simulink model "Helicopter_Non_linear_ex"  (R2018a)
settings: Solver=FixedStepAuto  StartTime=4371.0  StopTime=5862  FixedStep=0.2  RelTol=1e-3
model workspace (MAT data in the model file):
  tp6fc6b471_771e_48c6_9efd_2679798d0b46.time = 0
  tp6fc6b471_771e_48c6_9efd_2679798d0b46.signals(1).values = -0.785398163397
  tp6fc6b471_771e_48c6_9efd_2679798d0b46.signals(1).dimensions = 1
  tp6fc6b471_771e_48c6_9efd_2679798d0b46.signals(1).label = 'CSTATE'
  tp6fc6b471_771e_48c6_9efd_2679798d0b46.signals(1).blockName = 'Helicopter_Non_linear_ex/Integrator'
  tp6fc6b471_771e_48c6_9efd_2679798d0b46.signals(1).stateName = ''
  tp6fc6b471_771e_48c6_9efd_2679798d0b46.signals(1).inReferencedModel = 0
  tp6fc6b471_771e_48c6_9efd_2679798d0b46.signals(1).sampleTime = [0 0]
  tp6fc6b471_771e_48c6_9efd_2679798d0b46.signals(2).values = 1.21691147844
  tp6fc6b471_771e_48c6_9efd_2679798d0b46.signals(2).dimensions = 1
  tp6fc6b471_771e_48c6_9efd_2679798d0b46.signals(2).label = 'CSTATE'
  tp6fc6b471_771e_48c6_9efd_2679798d0b46.signals(2).blockName = 'Helicopter_Non_linear_ex/Integrator1'
  tp6fc6b471_771e_48c6_9efd_2679798d0b46.signals(2).stateName = ''
  tp6fc6b471_771e_48c6_9efd_2679798d0b46.signals(2).inReferencedModel = 0
  tp6fc6b471_771e_48c6_9efd_2679798d0b46.signals(2).sampleTime = [0 0]
  tp6fc6b471_771e_48c6_9efd_2679798d0b46.signals(3).values = 1
  tp6fc6b471_771e_48c6_9efd_2679798d0b46.signals(3).dimensions = 1
  tp6fc6b471_771e_48c6_9efd_2679798d0b46.signals(3).label = 'CSTATE'
  tp6fc6b471_771e_48c6_9efd_2679798d0b46.signals(3).blockName = 'Helicopter_Non_linear_ex/Integrator2'
  tp6fc6b471_771e_48c6_9efd_2679798d0b46.signals(3).stateName = ''
  tp6fc6b471_771e_48c6_9efd_2679798d0b46.signals(3).inReferencedModel = 0
  tp6fc6b471_771e_48c6_9efd_2679798d0b46.signals(3).sampleTime = [0 0]
  tp6fc6b471_771e_48c6_9efd_2679798d0b46.signals(4).values = -0.483892496659
  tp6fc6b471_771e_48c6_9efd_2679798d0b46.signals(4).dimensions = 1
  tp6fc6b471_771e_48c6_9efd_2679798d0b46.signals(4).label = 'CSTATE'
  tp6fc6b471_771e_48c6_9efd_2679798d0b46.signals(4).blockName = 'Helicopter_Non_linear_ex/Integrator3'
  tp6fc6b471_771e_48c6_9efd_2679798d0b46.signals(4).stateName = ''
  tp6fc6b471_771e_48c6_9efd_2679798d0b46.signals(4).inReferencedModel = 0
  tp6fc6b471_771e_48c6_9efd_2679798d0b46.signals(4).sampleTime = [0 0]
  tp898a3b84_44fb_438a_a53f_dc007c783af6.time = 310
  tp898a3b84_44fb_438a_a53f_dc007c783af6.signals(1).values = -4.83010382755
  tp898a3b84_44fb_438a_a53f_dc007c783af6.signals(1).dimensions = 1
  tp898a3b84_44fb_438a_a53f_dc007c783af6.signals(1).label = 'CSTATE'
  tp898a3b84_44fb_438a_a53f_dc007c783af6.signals(1).blockName = 'Helicopter_Non_linear_ex/Integrator'
  tp898a3b84_44fb_438a_a53f_dc007c783af6.signals(1).stateName = ''
  tp898a3b84_44fb_438a_a53f_dc007c783af6.signals(1).inReferencedModel = 0
  tp898a3b84_44fb_438a_a53f_dc007c783af6.signals(1).sampleTime = [0 0]
  tp898a3b84_44fb_438a_a53f_dc007c783af6.signals(2).values = 1.21691147844
  tp898a3b84_44fb_438a_a53f_dc007c783af6.signals(2).dimensions = 1
  tp898a3b84_44fb_438a_a53f_dc007c783af6.signals(2).label = 'CSTATE'
  tp898a3b84_44fb_438a_a53f_dc007c783af6.signals(2).blockName = 'Helicopter_Non_linear_ex/Integrator1'
  tp898a3b84_44fb_438a_a53f_dc007c783af6.signals(2).stateName = ''
  tp898a3b84_44fb_438a_a53f_dc007c783af6.signals(2).inReferencedModel = 0
  tp898a3b84_44fb_438a_a53f_dc007c783af6.signals(2).sampleTime = [0 0]
  tp898a3b84_44fb_438a_a53f_dc007c783af6.signals(3).values = 4.83651296756
  tp898a3b84_44fb_438a_a53f_dc007c783af6.signals(3).dimensions = 1
  tp898a3b84_44fb_438a_a53f_dc007c783af6.signals(3).label = 'CSTATE'
  tp898a3b84_44fb_438a_a53f_dc007c783af6.signals(3).blockName = 'Helicopter_Non_linear_ex/Integrator2'
  tp898a3b84_44fb_438a_a53f_dc007c783af6.signals(3).stateName = ''
  tp898a3b84_44fb_438a_a53f_dc007c783af6.signals(3).inReferencedModel = 0
  tp898a3b84_44fb_438a_a53f_dc007c783af6.signals(3).sampleTime = [0 0]
  tp898a3b84_44fb_438a_a53f_dc007c783af6.signals(4).values = -0.483892496659
  tp898a3b84_44fb_438a_a53f_dc007c783af6.signals(4).dimensions = 1
  tp898a3b84_44fb_438a_a53f_dc007c783af6.signals(4).label = 'CSTATE'
  tp898a3b84_44fb_438a_a53f_dc007c783af6.signals(4).blockName = 'Helicopter_Non_linear_ex/Integrator3'
  tp898a3b84_44fb_438a_a53f_dc007c783af6.signals(4).stateName = ''
  tp898a3b84_44fb_438a_a53f_dc007c783af6.signals(4).inReferencedModel = 0
  tp898a3b84_44fb_438a_a53f_dc007c783af6.signals(4).sampleTime = [0 0]
values from neighbouring files (symbols this model uses):
  Bp = 0.01    [Helicopter_Values.m]
  By = 0.08    [Helicopter_Values.m]
  g = 9.81    [Helicopter_Values.m]
  jeqp = 0.0172    [Helicopter_Values.m]
  jeqy = 0.021    [Helicopter_Values.m]
  kpp = 0.0556    [Helicopter_Values.m]
  kpy = 0.005    [Helicopter_Values.m]
  kyp = 0.15    [Helicopter_Values.m]
  kyy = 0.21084    [Helicopter_Values.m]
  lcm = 0.015    [Helicopter_Values.m]
  mheli = 0.479    [Helicopter_Values.m]
undefined symbols (not defined in the file or in its folder): d2r
settings Model: Creator=pacoa  LastModifiedBy=pacoa
settings DataIOCC: ExternalInput=tp035601c0_6253_4429_837b_fd395f9a609e(1),tp035601c0_6253_4429_837b_fd395f9a609e(2),tp035601c0_6253_4429_837b_fd395f9a609e(3),tp035601c0_6253_4429_837b_fd395f9a609e(4),tp035601c0_6253_4429_837b_fd395f9a609e(5),tp035601c0_6253_4429_837b_fd395f9a609e(6)  InitialState=tp6fc6b471_771e_48c6_9efd_2679798d0b46  ReturnWorkspaceOutputs=on  OutputOption=AdditionalOutputTimes  OutputTimes=SDO_OutputTimes  ReturnWorkspaceOutputsName=SDOSimTest_Log

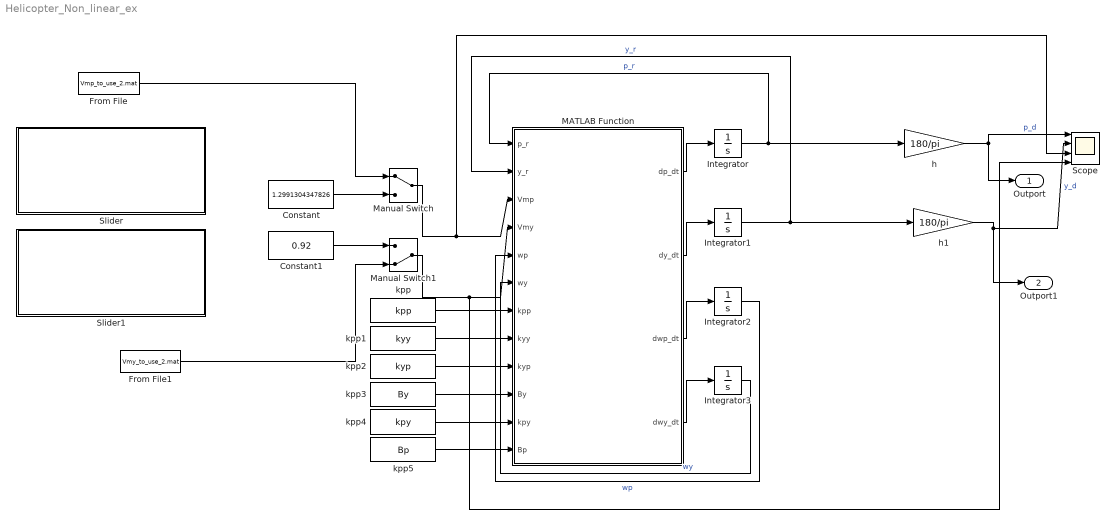
== system Helicopter_Non_linear_ex ==
  Constant : Constant  Value=1.2991304347826
  Constant1 : Constant  Value=0.92
  From File : FromFile  FileName=Vmp_to_use_2.mat  SampleTime=0.2  ExtrapolationBeforeFirstDataPoint=Hold first value  ExtrapolationAfterLastDataPoint=Hold last value
  From File1 : FromFile  FileName=Vmy_to_use_2.mat  SampleTime=0.2  ExtrapolationBeforeFirstDataPoint=Hold first value  ExtrapolationAfterLastDataPoint=Hold last value
  Integrator : Integrator  InitialCondition=d2r(-38.4107171239704)  LimitOutput=on  UpperSaturationLimit=pi/4  LowerSaturationLimit=-pi/4
  Integrator1 : Integrator  InitialCondition=d2r(79.0074564933032)  LimitOutput=on  UpperSaturationLimit=pi  LowerSaturationLimit=0
  Integrator2 : Integrator  LimitOutput=on  UpperSaturationLimit=1  LowerSaturationLimit=-1
  Integrator3 : Integrator
  MATLAB Function : MATLAB Function  TreatAsAtomicUnit=on
  Manual Switch : ManualSwitch
  Manual Switch1 : ManualSwitch  CurrentSetting=0
  Scope : Scope  NumInputPorts=4
  Slider : Subsystem  DialogController=hmiCreateDDGDialog  IsWebBlock=on  mask(MWDashboardBlock){webBlockId=04463d73-d6a9-4b3d-abfe-2f563ab264e6, webBlockType=slider, ShowInLibBrowser=on, ShowInitialText=on, HMISrcModelName=Helicopter_Non_linear_ex}
      mask prompts: webBlockId "WebBlock Id"; webBlockType "WebBlock Type"; HMISrcModelName "Source Model"
      mask help: SimulinkHMI:dialogs:SliderDialogDesc
      mask Help: helpview([docroot '/mapfiles/simulink.map'], 'hmi_slider')
      mask Display:
      | if strcmp(get_param(bdroot(gcb),'BlockDiagramType'), 'library')
      |     image([(matlabroot) '/toolbox/simulink/hmi/icons/Slider.png']);
      | end
  Slider1 : Subsystem  DialogController=hmiCreateDDGDialog  IsWebBlock=on  mask(MWDashboardBlock){webBlockId=82fec370-2a65-419d-b4f2-61c4ae5ab55a, webBlockType=slider, ShowInLibBrowser=on, ShowInitialText=on, HMISrcModelName=Helicopter_Non_linear_ex}
      mask prompts: webBlockId "WebBlock Id"; webBlockType "WebBlock Type"; HMISrcModelName "Source Model"
      mask help: SimulinkHMI:dialogs:SliderDialogDesc
      mask Help: helpview([docroot '/mapfiles/simulink.map'], 'hmi_slider')
      mask Display:
      | if strcmp(get_param(bdroot(gcb),'BlockDiagramType'), 'library')
      |     image([(matlabroot) '/toolbox/simulink/hmi/icons/Slider.png']);
      | end
  h : Gain  Gain=180/pi
  h1 : Gain  Gain=180/pi
  kpp : Constant  Value=kpp
  kpp1 : Constant  Value=kyy
  kpp2 : Constant  Value=kyp
  kpp3 : Constant  Value=By
  kpp4 : Constant  Value=kpy
  kpp5 : Constant  Value=Bp
  Outport : Outport
  Outport1 : Outport  Port=2
  wires:
  MATLAB Function/1(dp_dt) -> Integrator/1
  MATLAB Function/4(dwy_dt) -> Integrator3/1
  MATLAB Function/3(dwp_dt) -> Integrator2/1
  MATLAB Function/2(dy_dt) -> Integrator1/1
  Integrator/1 -> h/1, MATLAB Function/1(p_r)  "p_r"
  Integrator1/1 -> MATLAB Function/2(y_r), h1/1  "y_r"
  Integrator3/1 -> MATLAB Function/6(wy)  "wy"
  Integrator2/1 -> MATLAB Function/5(wp)  "wp"
  Manual Switch/1 -> Scope/3, MATLAB Function/3(Vmp)
  From File/1 -> Manual Switch/1
  From File1/1 -> Manual Switch1/2
  Manual Switch1/1 -> Scope/4, MATLAB Function/4(Vmy)
  h/1 -> Scope/1, Outport/1  "p_d"
  h1/1 -> Scope/2, Outport1/1  "y_d"
  Constant/1 -> Manual Switch/2
  Constant1/1 -> Manual Switch1/1
  kpp/1 -> MATLAB Function/7(kpp)
  kpp1/1 -> MATLAB Function/8(kyy)
  kpp2/1 -> MATLAB Function/9(kyp)
  kpp3/1 -> MATLAB Function/10(By)
  kpp4/1 -> MATLAB Function/11(kpy)
  kpp5/1 -> MATLAB Function/12(Bp)

== system Helicopter_Non_linear_ex/Slider ==

== system Helicopter_Non_linear_ex/Slider1 ==

== matlab function Helicopter_Non_linear_ex/MATLAB Function ==
  data: p_r input; y_r input; Vmp input; Vmy input; wp input; dp_dt output size=[1 1]; wy input; dy_dt output size=[1 1]; dwp_dt output size=[1 1]; dwy_dt output size=[1 1]; lcm parameter; mheli parameter; jeqp parameter; jeqy parameter; g parameter; kpp input; kyy input; kyp input; By input; kpy input; Bp input
function [dp_dt, dy_dt, dwp_dt, dwy_dt]= fcn(p_r,y_r,Vmp, Vmy,wp,wy, lcm, mheli, jeqp, jeqy, g, kpp, kyy, kyp, By, kpy, Bp)

  %%Parameters
%   
%   Bp,
%   By,
%   g,
%   kpp,
%   kyp,
%   kyy,
%   kpy,
%   mheli,
%   lcm,
%   jeqp,
%   jeqy,
  

%%
   dp_dt = wp;
   dy_dt = wy;
   
   %%
   dwp_dt_n1 = (kpp*Vmp);
   dwp_dt_n2 = (kpy*Vmy);
   dwp_dt_n3 = (Bp*wp+ (mheli*(wy.^2)*sin(p_r)*(lcm^2)*cos(p_r) + (mheli*g*cos(p_r)*lcm)));
   
   dwp_dt_d = (jeqp + mheli*(lcm^2));
   
   dwp_dt = (dwp_dt_n1 -dwp_dt_n2 - dwp_dt_n3)/(dwp_dt_d);
   
   %%
   dwy_dt_n1 = kyp*Vmp;
   dwy_dt_n2 = kyy*Vmy;
   dwy_dt_n3 = 2*mheli*(wy)*sin(p_r)*(lcm^2)*cos(p_r)*wp;
   dwy_dt_n4 = By*wy;
   
   dwy_dt_d = jeqy + mheli*((cos(p_r))^2)*(lcm^2);
   
   dwy_dt = (dwy_dt_n1 - dwy_dt_n2 + dwy_dt_n3 -dwy_dt_n4)/(dwy_dt_d);
